simulink library "lib_isae_drones"  (R2017b)
settings: Solver=ode45  StartTime=0.0  StopTime=10.0  RelTol=1e-3  EnableMultiTasking=on
undefined symbols (not defined in the file or in its folder): C_trainee, Imoteur, motor
libraries: drones x1
settings Model: Creator=f.defay  LastModifiedBy=f.defay
settings DataIOCC: LimitDataPoints=on  SaveFormat=StructureWithTime
settings OptimizationCC: LifeSpan=inf
settings DebuggingCC: AllowSymbolicDim=off  SFUnexpectedBacktrackingDiag=warning  SFNoUnconditionalDefaultTransitionDiag=warning  SFExecutionAtInitializationDiag=none
settings HardwareCC: ProdBitPerSizeT=32  ProdBitPerPtrDiffT=32  ProdWordSize=32  ProdHWDeviceType=Specified
settings ModelReferenceCC: PropagateSignalLabelsOutOfModel=off
settings CodeAppCC: StateflowObjectComments=on
settings GRTTargetCC: TargetLangStandard=C89/C90 (ANSI)
settings ConfigComp: CovMetricSettings=dw  CovHtmlReporting=on  CovSaveCumulativeToWorkspaceVar=on  CovSaveSingleToWorkspaceVar=on  CovExternalEMLEnable=off

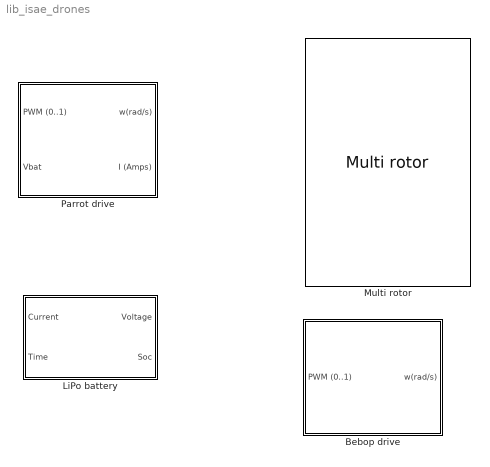
== system lib_isae_drones ==
  Bebop drive : Subsystem  mask{Time_constant=motor.tr_mot, coef_pwm2w=motor.coef_w2I, omega_0=motor.w0, omega_max=motor.wmax}
      mask prompts: Time_constant "Close loop Time constant (s)"; coef_pwm2w "Static gain"; omega_0 "Initial rotationnal speed (rad/s)"; omega_max "Maximal rotationnal Speed (rad/s)"
  LiPo battery : Subsystem  mask{nb_elements=3, capacity=1.5, initial_voltage=12.5, internal_resistance=0}
      mask prompts: nb_elements "Number of LiPo Elements"; capacity "Total Capacity of battery (Ah)"; initial_voltage "Initial Voltage at start"; internal_resistance "internal resistance"
      mask Display:
      | port_label('output', 1, 'voltage')
      | port_label('output', 2, 'soc')
      | port_label('input', 1, 'current')
      | port_label('input', 2, 'time')
      | disp('LiPo Battery')
  Multi rotor : drones/Multi rotor  thrust_factor=Pw  torque_coef=Mw  density=rho  drag_coef=C_trainee(1)*3  rotor_inertia=Imoteur(1,1)  prop_diameter=0.2  total_mass=mtot  aircraft_diameter=0.5  aircraft_type=1
  Parrot drive : Subsystem  mask{Time_constant=motor.tr_mot, coef_t2w=motor.coef_t2w, coef_curve=motor.coef_w2I, omega_0=motor.w0, omega_max=motor.wmax, V_nom=motor.nominal_voltage}
      mask prompts: Time_constant "Close loop Time constant (s)"; coef_t2w "PWM polynomial curve"; coef_curve "Polynomial coefficient for relation between the rotrionnal speed of the propeller and the current"; omega_0 "Initial rotationnal speed (rad/s)"; omega_max "Maximal rotationnal Speed (rad/s)"; V_nom "Nominal Motor Voltage (Volt)"

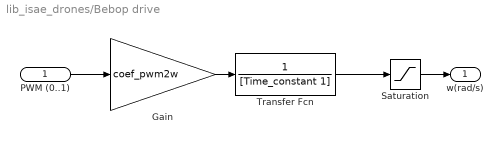
== system lib_isae_drones/Bebop drive ==
  PWM (0..1) : Inport  OutDataTypeStr=double  PortDimensions=1  SampleTime=0
  Gain : Gain  Gain=coef_pwm2w
  Saturation : Saturate  UpperLimit=omega_max  LowerLimit=0
  Transfer Fcn : TransferFcn  Denominator=[Time_constant 1]
  w(rad/s) : Outport  OutDataTypeStr=double  PortDimensions=1  SampleTime=0
  wires:
  Saturation/1 -> w(rad/s)/1
  Gain/1 -> Transfer Fcn/1
  Transfer Fcn/1 -> Saturation/1
  PWM (0..1)/1 -> Gain/1

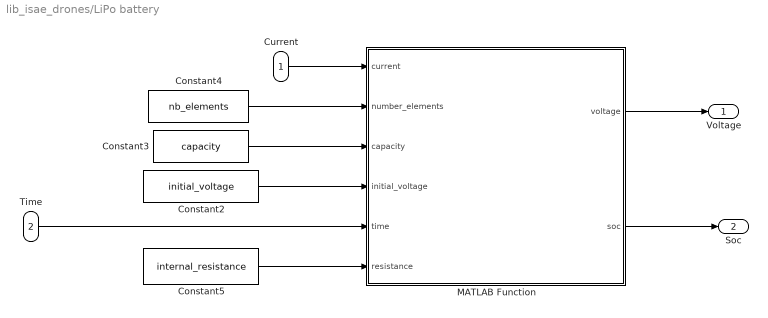
== system lib_isae_drones/LiPo battery ==
  Current : Inport
  Time : Inport  Port=2
  Constant2 : Constant  Value=initial_voltage
  Constant3 : Constant  Value=capacity
  Constant4 : Constant  Value=nb_elements
  Constant5 : Constant  Value=internal_resistance
  MATLAB Function : MATLAB Function  TreatAsAtomicUnit=on
  Voltage : Outport
  Soc : Outport  Port=2
  wires:
  Constant3/1 -> MATLAB Function/3(capacity)
  Constant2/1 -> MATLAB Function/4(initial_voltage)
  MATLAB Function/1(voltage) -> Voltage/1
  Constant4/1 -> MATLAB Function/2(number_elements)
  Constant5/1 -> MATLAB Function/6(resistance)
  Time/1 -> MATLAB Function/5(time)
  MATLAB Function/2(soc) -> Soc/1
  Current/1 -> MATLAB Function/1(current)

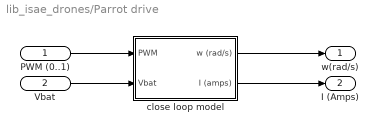
== system lib_isae_drones/Parrot drive ==
  PWM (0..1) : Inport  OutDataTypeStr=double  PortDimensions=1  SampleTime=0
  Vbat : Inport  Port=2  OutDataTypeStr=double  PortDimensions=1  SampleTime=0
  close loop model : Subsystem
  w(rad/s) : Outport  OutDataTypeStr=double  PortDimensions=1  SampleTime=0
  I (Amps) : Outport  Port=2  OutDataTypeStr=double  PortDimensions=1  SampleTime=0
  wires:
  close loop model/2(I (amps)) -> I (Amps)/1
  close loop model/1(w (rad/s)) -> w(rad/s)/1
  Vbat/1 -> close loop model/2("Vbat ")
  PWM (0..1)/1 -> close loop model/1(PWM)

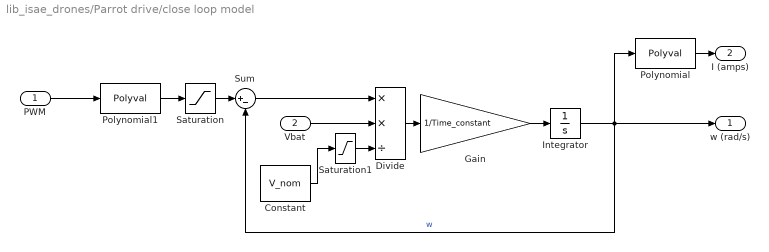
== system lib_isae_drones/Parrot drive/close loop model ==
  PWM : Inport
  "Vbat " : Inport  Port=2  OutDataTypeStr=double  PortDimensions=1  SampleTime=0
  Constant : Constant  Value=V_nom
  Divide : Product  Inputs=**/
  Gain : Gain  Gain=1/Time_constant
  Integrator : Integrator  InitialCondition=omega_0  LowerSaturationLimit=0
  Polynomial : Polyval  Coefs=coef_curve
  Polynomial1 : Polyval  Coefs=coef_t2w
  Saturation : Saturate  UpperLimit=omega_max  LowerLimit=0
  Saturation1 : Saturate  UpperLimit=100  LowerLimit=1
  Sum : Sum  Inputs=|+-
  w (rad/s) : Outport
  I (amps) : Outport  Port=2
  wires:
  Integrator/1 -> Polynomial/1, Sum/2, w (rad/s)/1  "w"
  Gain/1 -> Integrator/1
  "Vbat "/1 -> Divide/2
  PWM/1 -> Polynomial1/1
  Sum/1 -> Divide/1
  Divide/1 -> Gain/1
  Polynomial1/1 -> Saturation/1
  Polynomial/1 -> I (amps)/1
  Saturation/1 -> Sum/1
  Constant/1 -> Saturation1/1
  Saturation1/1 -> Divide/3

== matlab function lib_isae_drones/LiPo battery/MATLAB Function ==
  data: current input; voltage output; number_elements input; capacity input; initial_voltage input; time input; soc output; resistance input
function [voltage,soc] = battery_estimation(current,number_elements,capacity,initial_voltage,time,resistance)
%#Very simple model of LiPo Battery for simulation purpose.
% The model is completely linear and don'yttake account of the non
% linearity of the battery
%
% Input:
% Current : Actual current consumed (Amps)
% number_elements: Number elements of LiPo

nominal_element_voltage = 3.74;
maximal_element_voltage = 4.2;
minimal_element_volatge = 3.4;

persistent cell_voltage;
persistent initial_soc;
persistent actual_soc;
persistent time_of_use;
persistent last_time;
persistent initial_time;
persistent init;


if isempty(initial_soc)
    initial_soc = (initial_voltage/number_elements - minimal_element_volatge)/(maximal_element_voltage-minimal_element_volatge)*capacity;;
end
if isempty(actual_soc)
    actual_soc = initial_soc;
end
if isempty(cell_voltage)
    cell_voltage = initial_voltage/number_elements;
end
if isempty(time_of_use)
    time_of_use = 0;
end
if isempty(last_time)
    last_time = 0;
end
if isempty(initial_time)
    initial_time = time;
end


time_of_use = time - initial_time;
actual_soc = actual_soc - current * (time - last_time)/3600;

if (actual_soc < 0.25 * capacity)
    actual_soc = actual_soc - current * (time - last_time)/3600;
end

discharge_capacity = 1 - actual_soc/capacity;

cell_voltage = maximal_element_voltage-0.1 - 0.6 * discharge_capacity;

if ( discharge_capacity <=0.10 )
    cell_voltage = cell_voltage + (0.1-discharge_capacity)*(0.1-discharge_capacity)*(0.1-discharge_capacity) * 100;
elseif (discharge_capacity > 0.80)
    cell_voltage = cell_voltage - (discharge_capacity-0.8)*(discharge_capacity-0.8)*(discharge_capacity-0.8) * 50;
end

cell_voltage = cell_voltage - resistance * current;

last_time = time;
voltage = cell_voltage * number_elements - resistance * current;
soc = discharge_capacity;%actual_soc/capacity*100;
